simulink model "Instruction_decoder"  (R2021a)
settings: Solver=VariableStepAuto  StartTime=0.0  StopTime=inf  RelTol=1e-3
settings Model: Creator=kbhar  LastModifiedBy=kbhar

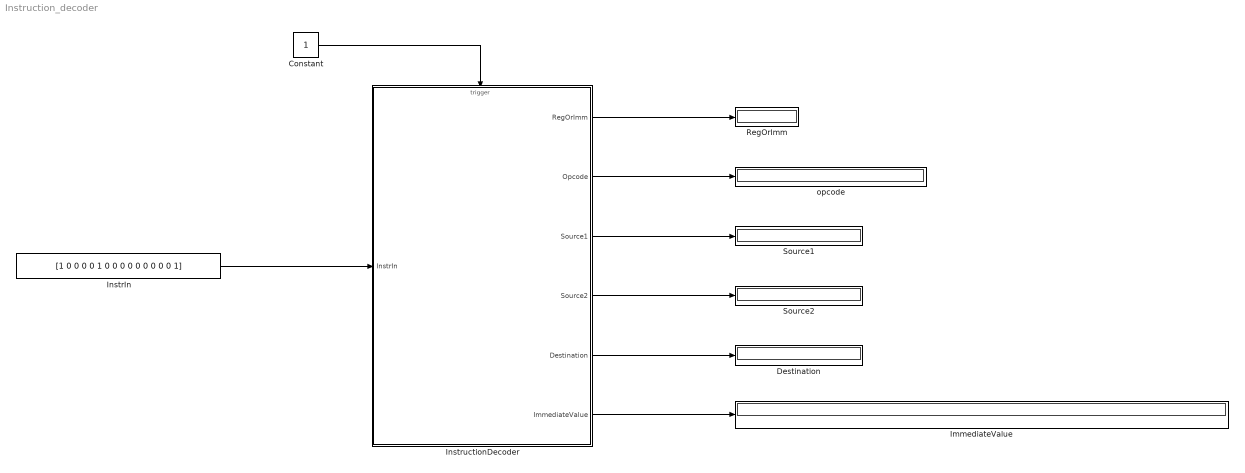
== system Instruction_decoder ==
  Constant : Constant
  Destination : Display
  ImmediateValue : Display
  "InstrIn " : Constant  Value=[1 0 0 0 0 1 0 0 0 0 0 0 0 0 0 1]
  InstructionDecoder : Subsystem
  RegOrImm : Display
  Source1 : Display
  Source2 : Display
  opcode : Display
  wires:
  "InstrIn "/1 -> InstructionDecoder/1(InstrIn)
  InstructionDecoder/6(ImmediateValue) -> ImmediateValue/1
  InstructionDecoder/5(Destination) -> Destination/1
  InstructionDecoder/4(Source2) -> Source2/1
  InstructionDecoder/3(Source1) -> Source1/1
  InstructionDecoder/2(Opcode) -> opcode/1
  InstructionDecoder/1(RegOrImm) -> RegOrImm/1
  Constant/1 -> InstructionDecoder/Trigger

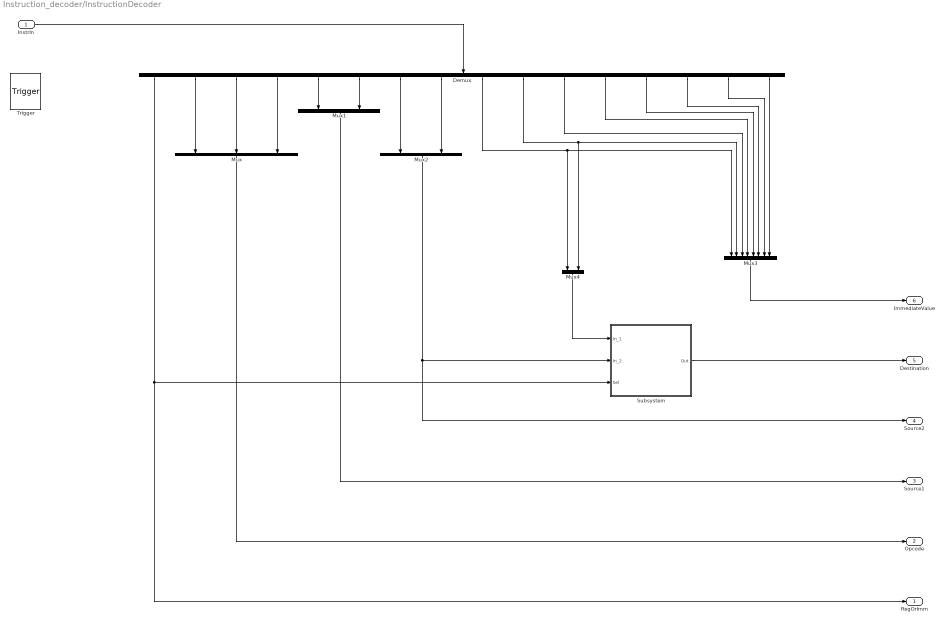
== system Instruction_decoder/InstructionDecoder ==
  InstrIn : Inport
  Trigger : TriggerPort  VariantControl=(inherit)  PortDimensions=1
  Demux : Demux  Outputs=16
  Mux : Mux  Inputs=3
  Mux1 : Mux  Inputs=2
  Mux2 : Mux  Inputs=2
  Mux3 : Mux  Inputs=8
  Mux4 : Mux  Inputs=2
  Subsystem : Subsystem
  RegOrImm : Outport
  Opcode : Outport  Port=2
  Source1 : Outport  Port=3
  Source2 : Outport  Port=4
  Destination : Outport  Port=5
  ImmediateValue : Outport  Port=6
  wires:
  Demux/4 -> Mux/3
  Mux4/1 -> Subsystem/1(In_1)
  Demux/12 -> Mux3/4
  Demux/9 -> Mux4/1, Mux3/1
  Demux/15 -> Mux3/7
  Demux/13 -> Mux3/5
  Demux/2 -> Mux/1
  Demux/14 -> Mux3/6
  Mux2/1 -> Source2/1, Subsystem/2(In_2)
  Demux/1 -> RegOrImm/1, Subsystem/3(Sel)
  Demux/6 -> Mux1/2
  Demux/5 -> Mux1/1
  Demux/7 -> Mux2/1
  Demux/8 -> Mux2/2
  Demux/10 -> Mux3/2, Mux4/2
  Demux/3 -> Mux/2
  Demux/16 -> Mux3/8
  Demux/11 -> Mux3/3
  Subsystem/1(Out) -> Destination/1
  Mux1/1 -> Source1/1
  InstrIn/1 -> Demux/1
  Mux3/1 -> ImmediateValue/1
  Mux/1 -> Opcode/1

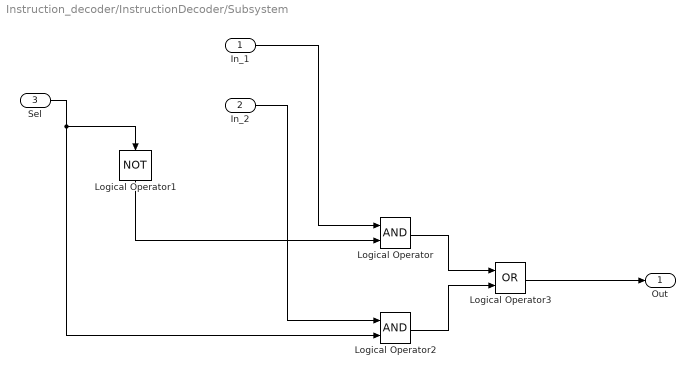
== system Instruction_decoder/InstructionDecoder/Subsystem ==
  In_1 : Inport
  In_2 : Inport  Port=2
  Sel : Inport  Port=3
  Logical Operator : Logic  AllPortsSameDT=off  OutDataTypeStr=boolean
  Logical Operator1 : Logic  Operator=NOT  AllPortsSameDT=off  OutDataTypeStr=boolean
  Logical Operator2 : Logic  AllPortsSameDT=off  OutDataTypeStr=boolean
  Logical Operator3 : Logic  Operator=OR  AllPortsSameDT=off  OutDataTypeStr=boolean
  Out : Outport
  wires:
  Logical Operator/1 -> Logical Operator3/1
  Logical Operator1/1 -> Logical Operator/2
  Sel/1 -> Logical Operator1/1, Logical Operator2/2
  Logical Operator2/1 -> Logical Operator3/2
  In_2/1 -> Logical Operator2/1
  In_1/1 -> Logical Operator/1
  Logical Operator3/1 -> Out/1
